simulink model "INTEGRATION_TEST_01"  (Simulink 8.1)
settings: Solver=ode4  StartTime=0.0  StopTime=inf  FixedStep=Ts  MaxStep=1e-3  RelTol=1e-3
model workspace (MAT data in the model file):
  op_snapshot1 : opcond.OperatingPoint (value not decoded)
PostLoadFcn:
  | INTEGRATION_TEST_01_init;
InitFcn:
  | INTEGRATION_TEST_01_init;
values from neighbouring files (symbols this model uses):
  SIM_HIL = 0    [INTEGRATION_TEST_01_init.m]
  Ts = 100E-6    (= 0.0001)    [INTEGRATION_TEST_01_init.m]
undefined symbols (not defined in the file or in its folder): cable_spec, cb_mech_delay, fdesignblkfcn, gcbh, Left, NG_CHP, NG_CHP_lib, ph, relay_par, type, V
libraries: simulink x23, rtio_opalrt_common x21, rtlab x7, simulink_extras x7, cables_lib x6, breaker_lib x4, rteventslib x4, Load_lib x3, rtio_generic_modbus x3, powerlib x2, ssn_lib x2, transformer_lib x2
(part 1 of 2)
settings Model: ARTEMISmethode_block_infos=$$__separator__$$INTEGRATION_TEST_01/ARTEMIS Guide$$__separator__$$  Creator=RE25624  LastModifiedBy=re25624  BufferReuse=off
settings SolverCC: ZeroCrossAlgorithm=Adaptive
settings DataIOCC: ExternalInput=getinputstruct(op_snapshot1)  InitialState=getstatestruct(op_snapshot1)  LimitDataPoints=off  MaxDataPoints=90060  SignalLoggingSaveFormat=Dataset  SaveOutput=off  SignalLogging=off  DSMLogging=off  SaveTime=off  OutputSaveName=result
settings OptimizationCC: BlockReduction=off  OptimizeBlockIOStorage=off  BufferReuse=off  ExpressionFolding=off  LocalBlockOutputs=off
settings DebuggingCC: MaxConsecutiveZCsMsg=warning  IgnoredZcDiagnostic=none  SolverPrmCheckMsg=none  MultiTaskRateTransMsg=warning  FcnCallInpInsideContextMsg=EnableAllAsWarning  FrameProcessingCompatibilityMsg=error  ModelReferenceExtraNoncontSigs=warning  StrictBusMsg=None
settings ModelReferenceCC: UpdateModelReferenceTargets=IfOutOfDate
settings SFSimCC: SFSimEcho=off
settings GRTTargetCC: CodeReplacementLibrary=C89/C90 (ANSI)

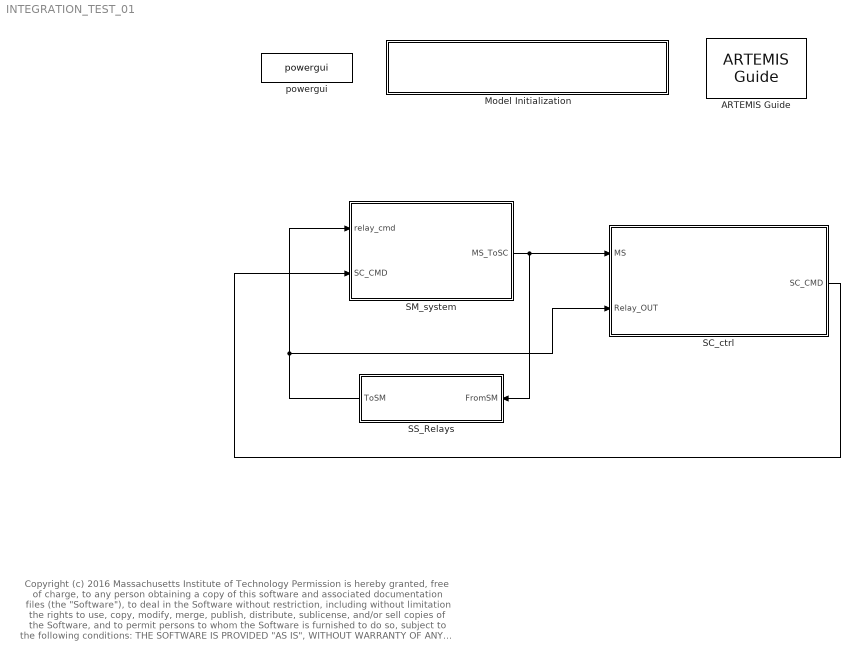
== system INTEGRATION_TEST_01 ==
  note: Copyright (c) 2016 Massachusetts Institute of Technology
      | Permission is hereby granted, free of charge, to any person obtaining a copy of this software and associated documentation files (the "Software"), to deal
      | in the Software without restriction, including without limitation the rights to use, copy, modify, merge, publish, distribute, sublicense, and/or sell copies of the
      | Software, and to permit persons to whom the Software is furnished to do so, subject to the following conditions:
      |
      | THE SOFTWARE IS PROVIDED "AS IS", WITHOUT WARRANTY OF ANY KIND, EXPRESS OR IMPLIED, INCLUDING BUT NOT LIMITED TO THE
      | WARRANTIES OF MERCHANTABILITY, FITNESS FOR A PARTICULAR PURPOSE AND NONINFRINGEMENT. IN NO EVENT SHALL THE AUTHORS
      | OR COPYRIGHT HOLDERS BE LIABLE FOR ANY CLAIM, DAMAGES OR OTHER LIABILITY, WHETHER IN AN ACTION OF CONTRACT, TORT OR
      | OTHERWISE, ARISING FROM, OUT OF OR IN CONNECTION WITH THE SOFTWARE OR THE USE OR OTHER DEALINGS IN THE SOFTWARE.
  ARTEMIS Guide : artemis/ARTEMIS/ARTEMIS Guide  Tag=FTSSmethode_opal_4hx0r99  Description=5.0_z1  lock=on  Ts=Ts  opt=art5  dyna=off  nb_perm=4  RT_fullcomp=off  ssn=on  ssn_itvc=off  ssn_ivic=off  ssn_ext=off  ssn_solver=Art5 with Backward Euler nodal interface  ssn_impulse=off  ssn_quasimpulse=off  ssn_impulse_loop=2  paraExtinctionThy=off  Thy_Impulse=on  dtc=Off  dtc_opt=normal  ao=on  simtype=off  ct_mac=off  lin_mov=off  lsp=[0.001 2]  spike_skip=Disabled  dtc_extra=1  dtc_sws=normal  dtc_pied=0.5  SPSRulesBlock=SPSRules  tre=on  ctmm=off  LF=off  dpl_type=ARTEMiS DPL  rlc_type=off  custom_type=off  para=on  ssn_ImpulseLoopBlockedStateUpdate=2  ssn_mov_iter_number=5  ssn_switch_iter_number=5
  Model Initialization : Subsystem  AncestorBlock=artemis/Tools /Misc/Model Initialization  mask(Model Functions){InitFcnX=INTEGRATION_TEST_01_init;, prel=off, posl=on, inif=on, strf=off}
      mask prompts: InitFcnX "Initialisation"; prel "Preload Function"; posl "PostLoad Function"; inif "InitFcn"; strf "StartFcn"
      mask init:
      | currentBlock = gcb;
      | root = bdroot(currentBlock);
      | 
      | 
      | if ~strcmp(get_param(root,'BlockDiagramType'),'library')
      |     if prel==1
      |         set_param(root, 'PreLoadFcn', InitFcnX);
      |     else
      |         set_param(root, 'PreLoadFcn', '');
      |     end
      |     if inif==1
      |         set_param(root, 'InitFcn', InitFcnX);
      |     else
      |         set_param(root, 'InitFcn', '');
      |     end
      |     if strf==1
      |         set_param(root, 'StartFcn', InitFcnX);
      |     else
      |         set_param(root, 'StartFcn', '');
      |     end
      |     if posl==1
      |         set_param(root, 'PostLoadFcn', InitFcnX);
      |     else
      |         set_param(root, 'PostLoadFcn', '');
      |     end
      | end
      | 
      | pos = get_param(currentBlock, 'Position');
      | width = pos(3) - pos(1); height = pos(4) - pos(2);
      | txt = [ upper(root) '\n' '- InitFcn. . . . . '  get_param(root, 'InitFcn') ];
      settings: CopyFcn=set_param(gcb,'LinkStatus','inactive')
      mask Display: text(5, height*0.5, txt, 'horizontalAlignment', 'left', 'verticalAlignment', 'middle') ;
  SC_ctrl : Subsystem
  SM_system : Subsystem
  SS_Relays : Subsystem
  powergui : powerlib/powergui  Priority=2  SimulationMode=Discrete  SolverType=Tustin  SampleTime=Ts  frequency=60  SPID=off  DisableSnubberDevices=off  DisableRonSwitches=off  DisableVfSwitches=off  SwTol=0  Interpol=off  DisplayEquations=off  frequencyindice=0  Pbase=100e6  ErrMax=1e-4  Iterations=50  UnitsV=kV  UnitsW=MW  FunctionMessages=off  echomessages=off  HookPort=off  EnableUseOfTLC=off  x0status=blocks  RestoreLinks=warning  ResistiveCurrentMeasurement=off  Frange=logspace(0,3,50)  Ylog=off  Xlog=off  ShowGrid=off  save=off  variable=ZData  structure=0  ZoomFFT=on  StartTime=0.0  cycles=2  DisplayStyle=off  fundamental=60  FreqAxis=off  MaxFrequency=1000  frequencyindicesteady=1  RmsSteady=1  display=off  Ts=0  methode=off
  wires:
  SM_system/1(MS_ToSC) -> SC_ctrl/1(MS), SS_Relays/1(FromSM)
  SS_Relays/1(ToSM) -> SM_system/1(relay_cmd), SC_ctrl/2(Relay_OUT)
  SC_ctrl/1(SC_CMD) -> SM_system/2(SC_CMD)

== system INTEGRATION_TEST_01/Model Initialization ==

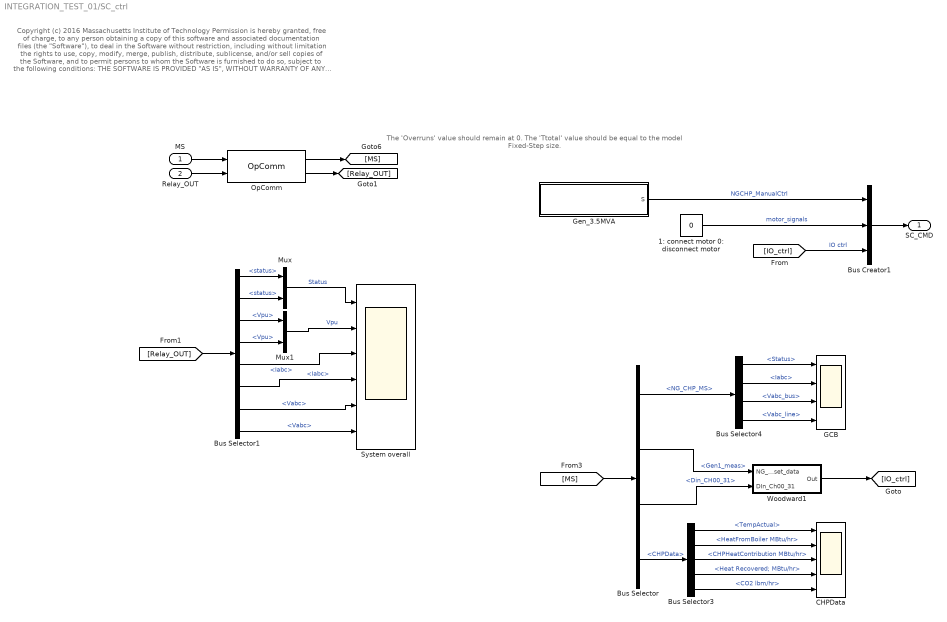
== system INTEGRATION_TEST_01/SC_ctrl ==
  note: The 'Overruns' value should remain at 0.
      | The 'Ttotal' value should be equal to the
      | model Fixed-Step size.
  note: Copyright (c) 2016 Massachusetts Institute of Technology
      | Permission is hereby granted, free of charge, to any person obtaining a copy of this software and associated documentation files (the "Software"), to deal
      | in the Software without restriction, including without limitation the rights to use, copy, modify, merge, publish, distribute, sublicense, and/or sell copies of the
      | Software, and to permit persons to whom the Software is furnished to do so, subject to the following conditions:
      |
      | THE SOFTWARE IS PROVIDED "AS IS", WITHOUT WARRANTY OF ANY KIND, EXPRESS OR IMPLIED, INCLUDING BUT NOT LIMITED TO THE
      | WARRANTIES OF MERCHANTABILITY, FITNESS FOR A PARTICULAR PURPOSE AND NONINFRINGEMENT. IN NO EVENT SHALL THE AUTHORS
      | OR COPYRIGHT HOLDERS BE LIABLE FOR ANY CLAIM, DAMAGES OR OTHER LIABILITY, WHETHER IN AN ACTION OF CONTRACT, TORT OR
      | OTHERWISE, ARISING FROM, OUT OF OR IN CONNECTION WITH THE SOFTWARE OR THE USE OR OTHER DEALINGS IN THE SOFTWARE
  MS : Inport
  Relay_OUT : Inport  Port=2
  1: connect motor 0: disconnect motor : Constant  Value=0
  Bus Creator1 : BusCreator  Inputs=3
  Bus Selector : BusSelector  OutputSignals=NG_CHP_MS,NG_CHP_MS.Gen1_meas,NG_CHP_MS.Din_CH00_31,NG_CHP_MS.CHPData
  Bus Selector1 : BusSelector  OutputSignals=CB2.m.status,CB3.m.status,CB2.m.Vpu,CB3.m.Vpu,CB2.m.Iabc,CB3.m.Iabc,CB2.m.Vabc,CB3.m.Vabc
  Bus Selector3 : BusSelector  OutputSignals=TempActual,HeatFromBoiler MBtu/hr,CHPHeatContribution MBtu/hr,Thermal data.Heat Recovered; MBtu/hr,Thermal data.CO2 lbm/hr
  Bus Selector4 : BusSelector  OutputSignals=NG_CHP_MS.Status,NG_CHP_MS.Iabc,NG_CHP_MS.Vabc_bus,NG_CHP_MS.Vabc_line
  CHPData : Scope  NumInputPorts=5
      settings: ShowLegends=on  TimeRange=10  YMin=20~0~-1~1.37518~932.98  YMax=20.05~5.5~1~1.37533~933.08  SaveName=ScopeData5
  GCB : Scope  NumInputPorts=4
      settings: ShowLegends=on  TimeRange=0.02  YMin=0.95~-800~-100000~-100000  YMax=1.05~800~130000~130000
  Gen_3.5MVA : Subsystem
  Mux : Mux  Inputs=2
  Mux1 : Mux  Inputs=2
  OpComm : rtlab/OpComm  nbport=2  groupe_acq=1  subsys_rate=0  st=0  Synchronization=on  Interpolation=on  Threshold=1.0  Missed_Data=off  Sim_Time=off  Samples=off  dynSigOut=off  from_console=0  warning_done=off  writeOpCommFile=off  Offset=off
  System overall : Scope  NumInputPorts=6
      settings: ShowLegends=on  TimeRange=1  YMin=0~0~-100~-200~-20000~-20000  YMax=5~1.5~100~200~20000~20000
  Woodward1 : Subsystem
  SC_CMD : Outport
  wires:
  OpComm/1 -> [MS]
  MS/1 -> OpComm/1
  OpComm/2 -> [Relay_OUT]
  Relay_OUT/1 -> OpComm/2
  Woodward1/1(Out) -> [IO_ctrl]
  Bus Selector4/1 -> GCB/1  "<Status>"
  Bus Selector4/2 -> GCB/2  "<Iabc>"
  Bus Selector4/3 -> GCB/3  "<Vabc_bus>"
  Bus Selector4/4 -> GCB/4  "<Vabc_line>"
  Bus Selector/1 -> Bus Selector4/1  "<NG_CHP_MS>"
  Bus Selector/2 -> Woodward1/1(NG_genset_data)  "<Gen1_meas>"
  Bus Selector/3 -> Woodward1/2(DIn_Ch00_31)  "<Din_CH00_31>"
  [MS] -> Bus Selector/1
  Bus Selector/4 -> Bus Selector3/1  "<CHPData>"
  Bus Selector3/1 -> CHPData/1  "<TempActual>"
  Bus Selector3/5 -> CHPData/5  "<CO2 lbm/hr>"
  Bus Selector3/2 -> CHPData/2  "<HeatFromBoiler MBtu/hr>"
  Bus Selector3/3 -> CHPData/3  "<CHPHeatContribution MBtu/hr>"
  Bus Selector3/4 -> CHPData/4  "<Heat Recovered; MBtu/hr>"
  [Relay_OUT] -> Bus Selector1/1
  Mux/1 -> System overall/1  "Status"
  Bus Selector1/1 -> Mux/1  "<status>"
  Bus Selector1/2 -> Mux/2  "<status>"
  Bus Selector1/3 -> Mux1/1  "<Vpu>"
  Bus Selector1/4 -> Mux1/2  "<Vpu>"
  Bus Selector1/5 -> System overall/3  "<Iabc>"
  Bus Selector1/6 -> System overall/4  "<Iabc>"
  Bus Selector1/7 -> System overall/5  "<Vabc>"
  Bus Selector1/8 -> System overall/6  "<Vabc>"
  Mux1/1 -> System overall/2  "Vpu"
  Bus Creator1/1 -> SC_CMD/1
  1: connect motor 0: disconnect motor/1 -> Bus Creator1/2  "motor_signals"
  [IO_ctrl] -> Bus Creator1/3  "IO ctrl"
  Gen_3.5MVA/1(S) -> Bus Creator1/1  "NGCHP_ManualCtrl"

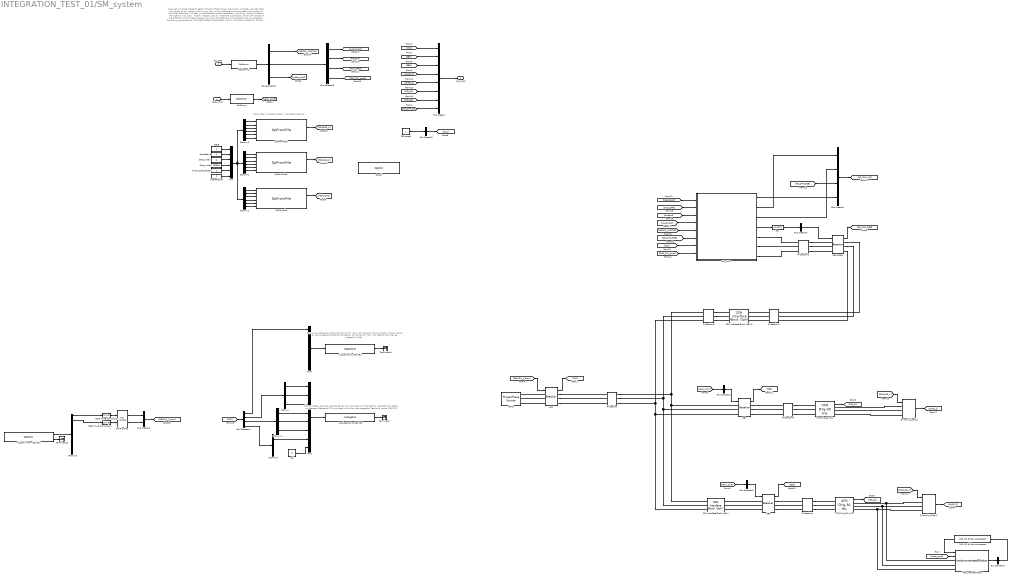
== system INTEGRATION_TEST_01/SM_system ==
  note: Copyright (c) 2016 Massachusetts Institute of Technology
      | Permission is hereby granted, free of charge, to any person obtaining a copy of this software and associated documentation files (the "Software"), to deal
      | in the Software without restriction, including without limitation the rights to use, copy, modify, merge, publish, distribute, sublicense, and/or sell copies of the
      | Software, and to permit persons to whom the Software is furnished to do so, subject to the following conditions:
      |
      | THE SOFTWARE IS PROVIDED "AS IS", WITHOUT WARRANTY OF ANY KIND, EXPRESS OR IMPLIED, INCLUDING BUT NOT LIMITED TO THE
      | WARRANTIES OF MERCHANTABILITY, FITNESS FOR A PARTICULAR PURPOSE AND NONINFRINGEMENT. IN NO EVENT SHALL THE AUTHORS
      | OR COPYRIGHT HOLDERS BE LIABLE FOR ANY CLAIM, DAMAGES OR OTHER LIABILITY, WHETHER IN AN ACTION OF CONTRACT, TORT OR
      | OTHERWISE, ARISING FROM, OUT OF OR IN CONNECTION WITH THE SOFTWARE OR THE USE OR OTHER DEALINGS IN THE SOFTWARE
  note: Stop_index = length of data - 1 to data chopping
  note: This connector also services Genset #2 and  is
      | shared with Genset #1.  Use RJ45 connectors to
      |  intercept Genset #2 I/O (not used in this Device
      | Integration Test) and use for SEL-751
  note: Remove existing connections to Slot 3 I/O, if any
      | ans replace with connections shown below, or use
      | corresponding RJ45 connectors.  (Existing I/O, if any not
      |  used for this Device Integration Test)
  relay_cmd : Inport
  SC_CMD : Inport  Port=2
  200 HP chiller compressor : Load_lib/200 HP chiller compressor
  AnalogOut2 to SEL-751 : rtio_opalrt_common/AnalogOut  CtrlName='OpCtrl'  portNb=4  FcnNos=Slot 2 Module A Subsection 2  size=16  maxcount=8  count=8  numchan=8  israngeinput=off  voltagerange=[ -5 ... 5 ]  slot=1  side=0  mismatch=0  slotside=Slot_2_Module_A
      settings: AttributesFormatString=%<CtrlName>
  Bus Creator : BusCreator  Inputs=8
  Bus Creator1 : BusCreator
  Bus Creator2 : BusCreator  Inputs=1
  Bus Creator3 : BusCreator  Inputs=1
  Bus Creator4 : BusCreator  Inputs=2
  Bus Selector1 : BusSelector  OutputSignals=CB2
  Bus Selector2 : BusSelector  OutputSignals=CB3
  Bus Selector3 : BusSelector  OutputSignals=NGCHP_ManualCtrl,IO ctrl,motor_signals
  Bus Selector4 : BusSelector  OutputSignals=Status,Iabc,Vabc_line,Vabc_bus
  Bus Selector5 : BusSelector  OutputSignals=Woodward,manual_controls,DOUT GR3,DOUT GR3.16 DOUT GR3.CHP_SIM_Cmds
  Bus Selector6 : BusSelector  OutputSignals=RPM
  CB closed : Constant
  CB1-GCB1 : breaker_lib/Breaker  Ts=Ts  mech_delays=[cb_mech_delay(1,:)]
  CB2 : breaker_lib/Breaker  Ts=Ts  mech_delays=[cb_mech_delay(1,:)]
  CB3 : breaker_lib/Breaker  Ts=Ts  mech_delays=[cb_mech_delay(1,:)]
  Cal : Constant  Value=0
  Data Type Conversion : DataTypeConversion
  Data Type Conversion1 : DataTypeConversion
  Demux : Demux  Outputs=3
  Demux1 : Demux  Outputs=6
  Demux2 : Demux  Outputs=6
  Demux3 : Demux  Outputs=6
  Demux4 : Demux  Outputs=3
  Demux5 : Demux  Outputs=3
  Demux6 : Demux  Outputs=8
  DigitalIn from SEL-751 : rtio_opalrt_common/DigitalIn  CtrlName='OpCtrl'  portNb=6  FcnNos=Slot 3 Module A Subsection 2  size=1  maxcount=8  count=8  sampleTime=Ts  numchan=8
      settings: AttributesFormatString=%<CtrlName>
  DigitalOut to SEL-751 : rtio_opalrt_common/DigitalOut  CtrlName='OpCtrl'  portNb=6  FcnNos=Slot 3 Module B Subsection 2  size=1  maxcount=8  count=8  numchan=8
      settings: AttributesFormatString=%<CtrlName>
  Dynamic_Load_1 : Load_lib/Dynamic_Load  V=4160  Ts=Ts
  Dynamic_Load_2 : Load_lib/Dynamic_Load  V=480  Ts=Ts
  Fcn : Fcn  Expr=u(1)==1
  GRID : powerlib/Electrical Sources/Three-Phase Source  Voltage=13800  PhaseAngle=0  Frequency=60  InternalConnection=Yg  SpecifyImpedance=on  Resistance=0.8929  Inductance=16.58e-3  ShortCircuitLevel=375e6  BaseVoltage=13800  XRratio=4.6  BusType=swing  Pref=0  Qref=0  Qmin=-inf  Qmax=inf
  InstrumentedMotor : Motor_InductionMachine_lib/InstrumentedMotor
  "Interpolation " : Constant
  MID : breaker_lib/Breaker  Ts=Ts  mech_delays=[cb_mech_delay(1,:)]
  Mux : Mux  Inputs=6
  Mux1 : Mux  Inputs=8
  Mux4 : Mux  Inputs=8
  NG_CHP1 : Subsystem  AncestorBlock=NG_CHP_lib/NG_CHP
  OpComm : rtlab/OpComm  nbport=1  groupe_acq=1  subsys_rate=0  st=0  Synchronization=on  Interpolation=on  Threshold=1.0  Missed_Data=off  Sim_Time=off  Samples=off  dynSigOut=off  from_console=0  warning_done=off  writeOpCommFile=off  Offset=off
  OpComm2 : rtlab/OpComm  nbport=1  groupe_acq=1  subsys_rate=0  st=0  Synchronization=on  Interpolation=on  Threshold=1.0  Missed_Data=off  Sim_Time=off  Samples=off  dynSigOut=off  from_console=1  warning_done=off  writeOpCommFile=off  Offset=off
  OpCtrl : rtio_opalrt_common/OpCtrl  CtrlName='OpCtrl'  boardid=0  BitstreamFilename=VC707_2-EX-0001-2_2_6_61-32AIO16DIO16DIOSel-01-01.bin  numconfig=-1  mode=Master  externalClock=off  decimRtsi=0  calibIO=off  SampleTime=0  loadinport=-1  BoardType=VC707  SecondaryPresent=off  sync_type=Audio
  OpFromFile : rtlab/DataLogging/OpFromFile  filename_mode=Static (same filename all the time)  reload_mode=Next time model is paused (Real-Time)  init_file_id=0  filename=HeatLoad.mat  rtpath='./'  nrtpath='.\'  sample_time=Ts
  OpFromFile1 : rtlab/DataLogging/OpFromFile  filename_mode=Static (same filename all the time)  reload_mode=Next time model is paused (Real-Time)  init_file_id=0  filename=one_min_data.mat  rtpath='./'  nrtpath='.\'  sample_time=0
  OpFromFile2 : rtlab/DataLogging/OpFromFile  filename_mode=Static (same filename all the time)  reload_mode=Next time model is paused (Real-Time)  init_file_id=0  filename=one_min_data.mat  rtpath='./'  nrtpath='.\'  sample_time=0
  PI-Section : cables_lib/PI-Section  cable_spec=[cable_spec(13, :)]  line_length=5500  parallel_sets=1
  PI-Section1 : cables_lib/PI-Section  cable_spec=[cable_spec(11, :)]  line_length=10  parallel_sets=1
  PI-Section2 : cables_lib/PI-Section  cable_spec=[cable_spec(11, :)]  line_length=2000  parallel_sets=1
  PI-Section3 : cables_lib/PI-Section  cable_spec=[cable_spec(13, :)]  line_length=1500  parallel_sets=1
  PI-Section4 : cables_lib/PI-Section  cable_spec=[cable_spec(13, :)]  line_length=7000  parallel_sets=1
  PI-Section5 : cables_lib/PI-Section  cable_spec=[cable_spec(11, :)]  line_length=10  parallel_sets=1
  "Repetative " : Constant
  S-R Flip-Flop : simulink_extras/Flip Flops/S-R Flip-Flop  initial_condition=1
  SSN Interface Block (3ph) : ssn_lib/SSN Interface Block (3ph)  nb_phase=3  nb_port=2  p1_type=V-type(Left)  p2_type=V-type (Right)  p3_type=V-type(Left)  p4_type=V-type(Left)  p5_type=V-type(Left)  p6_type=V-type(Left)  p7_type=V-type(Left)  p8_type=V-type(Left)  p9_type=V-type(Left)  p10_type=V-type(Left)  p11_type=V-type(Left)  p12_type=V-type(Left)  p13_type=V-type(Left)  p14_type=V-type(Left)  p15_type=V-type(Left)  p16_type=V-type(Left)  I_port_shunt_resistance=1e9
  SSN Interface Block (3ph)1 : ssn_lib/SSN Interface Block (3ph)  nb_phase=3  nb_port=2  p1_type=V-type(Left)  p2_type=V-type (Right)  p3_type=V-type(Left)  p4_type=V-type(Left)  p5_type=V-type(Left)  p6_type=V-type(Left)  p7_type=V-type(Left)  p8_type=V-type(Left)  p9_type=V-type(Left)  p10_type=V-type(Left)  p11_type=V-type(Left)  p12_type=V-type(Left)  p13_type=V-type(Left)  p14_type=V-type(Left)  p15_type=V-type(Left)  p16_type=V-type(Left)  I_port_shunt_resistance=1e9
  "Start_Index " : Constant
  "State " : Constant
  "Stop_Index " : Constant  Value=1800-1
  Terminator : Terminator
  Terminator1 : Terminator
  Terminator2 : Terminator
  "Time_Scale_Factor " : Constant
  XFR DYg-30 HIL1 : transformer_lib/XFR DYg-30 HIL  Rating=3750  Vp=13800  Vs=4160  Z=4.75  XR=11.4
  XFR DYg-30 HIL2 : transformer_lib/XFR DYg-30 HIL  Rating=2500  Vp=13800  Vs=480  Z=5.75  XR=6.6
  MS_ToSC : Outport
  wires:
  MID/1 -> [MID]
  Bus Creator/1 -> MS_ToSC/1
  OpComm/1 -> [relay_cmd]
  relay_cmd/1 -> OpComm/1
  CB1-GCB1/1 -> [NG_CHP_GCB]
  SC_CMD/1 -> OpComm2/1
  Bus Selector5/1 -> [woodward]  "<Woodward>"
  Bus Selector5/3 -> [Dout_GR3]  "<DOUT GR3>"
  Bus Selector5/2 -> [brkcont]  "<manual_controls>"
  [NG_CHP_GCB] -> Bus Creator1/3  "NG_CHP_MS"
  NG_CHP1/3(Generator Data) -> Bus Creator1/2  "Gen1_meas"
  NG_CHP1/2(Out2) -> Bus Creator1/1  "Din_CH00_31"
  XFR DYg-30 HIL1/1 -> [XFR_01]
  "Stop_Index "/1 -> Mux/4
  Demux1/2 -> OpFromFile1/2
  Demux1/5 -> OpFromFile1/5
  OpFromFile1/2 -> [PQLOAD_2]
  "Interpolation "/1 -> Mux/6
  Demux1/4 -> OpFromFile1/4
  Demux1/1 -> OpFromFile1/1
  Demux1/6 -> OpFromFile1/6
  Demux1/3 -> OpFromFile1/3
  "Start_Index "/1 -> Mux/3
  "Time_Scale_Factor "/1 -> Mux/5
  "Repetative "/1 -> Mux/2
  "State "/1 -> Mux/1
  [Dout_GR3] -> NG_CHP1/2(Digital Outputs)
  [brkcont] -> NG_CHP1/3(Console Breakers)
  [woodward] -> NG_CHP1/4(Woodward Enable)
  [NGCHP_MNCTLR] -> NG_CHP1/5(Manual Control (opt))
  [NG_CHP_GCB] -> NG_CHP1/6(GCB)
  [MID] -> NG_CHP1/7(MCB)
  NG_CHP1/1(Out1) -> Bus Creator1/4  "CHPData"
  NG_CHP1/4(GCB Control) -> Fcn/1
  Bus Selector5/4 -> [CHP_SIM_cmds]  "<CHP_SIM_Cmds>"
  OpFromFile/2 -> [heat_load]  "Heat Load MBtu/hr"
  [heat_load] -> NG_CHP1/1(In1)
  [CHP_SIM_cmds] -> NG_CHP1/8(In2)
  Demux2/2 -> OpFromFile/2
  Demux2/5 -> OpFromFile/5
  Demux2/4 -> OpFromFile/4
  Demux2/1 -> OpFromFile/1
  Demux2/6 -> OpFromFile/6
  Demux2/3 -> OpFromFile/3
  Dynamic_Load_1/1 -> [LOAD_1]
  XFR DYg-30 HIL2/1 -> [XFR_02]
  Dynamic_Load_2/1 -> [LOAD_2]
  Bus Creator2/1 -> [cb_c]
  CB closed/1 -> Bus Creator2/1  "Logic_trip"
  CB2/1 -> [CB2]
  CB3/1 -> [CB3]
  [XFR_02] -> Bus Creator/7  "XFR_02"
  [LOAD_2] -> Bus Creator/5  "LOAD_2"
  [XFR_01] -> Bus Creator/6  "XFR_01"
  [MID] -> Bus Creator/1  "MID"
  [CB3] -> Bus Creator/3  "CB3"
  [CB2] -> Bus Creator/2  "CB2"
  [LOAD_1] -> Bus Creator/4  "LOAD_1"
  Bus Creator1/1 -> [NG_CHP_MS]
  [NG_CHP_MS] -> Bus Creator/8  "NG_CHP_MS"
  Demux3/2 -> OpFromFile2/2
  Demux3/5 -> OpFromFile2/5
  OpFromFile2/2 -> [PQLOAD_1]
  Demux3/4 -> OpFromFile2/4
  Demux3/1 -> OpFromFile2/1
  Demux3/6 -> OpFromFile2/6
  Demux3/3 -> OpFromFile2/3
  Mux/1 -> Demux3/1, Demux2/1, Demux1/1
  [PQLOAD_1] -> Dynamic_Load_1/1
  [PQLOAD_2] -> Dynamic_Load_2/1
  [relay_cmd] -> Bus Selector1/1
  Bus Selector1/1 -> CB2/1  "<CB2>"
  [relay_cmd] -> Bus Selector2/1
  Bus Selector2/1 -> CB3/1  "<CB3>"
  Fcn/1 -> Bus Creator3/1  "Logic_trip"
  Bus Creator3/1 -> CB1-GCB1/1  "Logic_trip"
  [SEL751_1_from] -> MID/1
  [motor_cmd] -> InstrumentedMotor/2
  InstrumentedMotor/1 -> Bus Selector6/1
  Bus Selector6/1 -> 200 HP chiller compressor/1  "<RPM>"
  200 HP chiller compressor/1 -> InstrumentedMotor/1
  OpComm2/1 -> Bus Selector3/1
  Bus Selector3/1 -> [NGCHP_MNCTLR]  "<NGCHP_ManualCtrl>"
  Bus Selector3/2 -> Bus Selector5/1  "<IO ctrl>"
  Bus Selector3/3 -> [motor_cmd]  "<motor_signals>"
  Bus Selector4/2 -> Demux/1  "<Iabc>"
  Demux4/1 -> Mux1/4  "Va"
  Demux4/2 -> Mux1/5  "Vb"
  Demux4/3 -> Mux1/6  "Vc"
  Bus Selector4/4 -> Demux5/1  "<Vabc_bus>"
  Demux5/1 -> Mux1/7  "Vs"
  Bus Selector4/3 -> Demux4/1  "<Vabc_line>"
  Cal/1 -> Mux1/8
  AnalogOut2 to SEL-751/1 -> Terminator/1
  DigitalIn from SEL-751/1 -> Demux6/1
  Demux6/1 -> Data Type Conversion/1  "OUT103 Brkr trip"
  Demux6/2 -> Data Type Conversion1/1  "OUT102 Brkr reset"
  Data Type Conversion/1 -> S-R Flip-Flop/1
  Data Type Conversion1/1 -> S-R Flip-Flop/2
  S-R Flip-Flop/1 -> Bus Creator4/1  "Logic_trip"
  S-R Flip-Flop/2 -> Bus Creator4/2  "Logic_reset"
  Bus Selector4/1 -> Mux4/1  "<Status>"
  Mux4/1 -> DigitalOut to SEL-751/1
  DigitalOut to SEL-751/1 -> Terminator1/1
  DigitalIn from SEL-751/2 -> Terminator2/1
  Mux1/1 -> AnalogOut2 to SEL-751/1
  Demux/1 -> Mux1/1  "Ia"
  Demux/3 -> Mux1/3  "Ic"
  Demux/2 -> Mux1/2  "Ib"
  Bus Creator4/1 -> [SEL751_1_from]
  [MID] -> Bus Selector4/1
  connections:
  Dynamic_Load_1/LConn1 -- XFR DYg-30 HIL1/RConn1
  Dynamic_Load_1/LConn2 -- XFR DYg-30 HIL1/RConn2
  Dynamic_Load_1/LConn3 -- XFR DYg-30 HIL1/RConn3
  CB2/RConn2 -- PI-Section3/LConn2
  CB2/RConn1 -- PI-Section3/LConn1
  CB2/RConn3 -- PI-Section3/LConn3
  CB3/RConn2 -- PI-Section4/LConn2
  CB3/RConn1 -- PI-Section4/LConn1
  CB3/RConn3 -- PI-Section4/LConn3
  CB3/LConn2 -- SSN Interface Block (3ph)/RConn2
  CB3/LConn1 -- SSN Interface Block (3ph)/RConn1
  CB3/LConn3 -- SSN Interface Block (3ph)/RConn3
  PI-Section5/LConn3 -- PI-Section/RConn3 -- SSN Interface Block (3ph)/LConn3 -- CB2/LConn3
  PI-Section5/LConn2 -- PI-Section/RConn2 -- SSN Interface Block (3ph)/LConn2 -- CB2/LConn2
  PI-Section5/LConn1 -- PI-Section/RConn1 -- SSN Interface Block (3ph)/LConn1 -- CB2/LConn1
  Dynamic_Load_2/LConn1 -- InstrumentedMotor/LConn1 -- XFR DYg-30 HIL2/RConn1
  Dynamic_Load_2/LConn3 -- InstrumentedMotor/LConn3 -- XFR DYg-30 HIL2/RConn3
  Dynamic_Load_2/LConn2 -- InstrumentedMotor/LConn2 -- XFR DYg-30 HIL2/RConn2
  PI-Section4/RConn1 -- XFR DYg-30 HIL2/LConn1
  PI-Section4/RConn2 -- XFR DYg-30 HIL2/LConn2
  PI-Section4/RConn3 -- XFR DYg-30 HIL2/LConn3
  PI-Section3/RConn2 -- XFR DYg-30 HIL1/LConn2
  PI-Section3/RConn3 -- XFR DYg-30 HIL1/LConn3
  PI-Section3/RConn1 -- XFR DYg-30 HIL1/LConn1
  PI-Section2/RConn3 -- CB1-GCB1/LConn3
  PI-Section2/RConn2 -- CB1-GCB1/LConn2
  PI-Section2/RConn1 -- CB1-GCB1/LConn1
  NG_CHP1/RConn2 -- PI-Section2/LConn2
  NG_CHP1/RConn3 -- PI-Section2/LConn3
  NG_CHP1/RConn1 -- PI-Section2/LConn1
  PI-Section1/LConn1 -- SSN Interface Block (3ph)1/RConn1
  PI-Section1/LConn2 -- SSN Interface Block (3ph)1/RConn2
  PI-Section1/LConn3 -- SSN Interface Block (3ph)1/RConn3
  PI-Section5/RConn2 -- SSN Interface Block (3ph)1/LConn2
  PI-Section5/RConn1 -- SSN Interface Block (3ph)1/LConn1
  PI-Section5/RConn3 -- SSN Interface Block (3ph)1/LConn3
  CB1-GCB1/RConn3 -- PI-Section1/RConn3
  CB1-GCB1/RConn1 -- PI-Section1/RConn1
  CB1-GCB1/RConn2 -- PI-Section1/RConn2
  MID/RConn3 -- PI-Section/LConn3
  MID/RConn2 -- PI-Section/LConn2
  MID/RConn1 -- PI-Section/LConn1
  MID/LConn3 -- GRID/RConn3
  MID/LConn1 -- GRID/RConn1
  MID/LConn2 -- GRID/RConn2

== system INTEGRATION_TEST_01/SS_Relays ==
  note: Copyright (c) 2016 Massachusetts Institute of Technology
      | Permission is hereby granted, free of charge, to any person obtaining a copy of this software and associated documentation files (the "Software"), to deal
      | in the Software without restriction, including without limitation the rights to use, copy, modify, merge, publish, distribute, sublicense, and/or sell copies of the
      | Software, and to permit persons to whom the Software is furnished to do so, subject to the following conditions:
      |
      | THE SOFTWARE IS PROVIDED "AS IS", WITHOUT WARRANTY OF ANY KIND, EXPRESS OR IMPLIED, INCLUDING BUT NOT LIMITED TO THE
      | WARRANTIES OF MERCHANTABILITY, FITNESS FOR A PARTICULAR PURPOSE AND NONINFRINGEMENT. IN NO EVENT SHALL THE AUTHORS
      | OR COPYRIGHT HOLDERS BE LIABLE FOR ANY CLAIM, DAMAGES OR OTHER LIABILITY, WHETHER IN AN ACTION OF CONTRACT, TORT OR
      | OTHERWISE, ARISING FROM, OUT OF OR IN CONNECTION WITH THE SOFTWARE OR THE USE OR OTHER DEALINGS IN THE SOFTWARE
  FromSM : Inport
  Bus Creator : BusCreator  Inputs=2
  Bus Selector : BusSelector  OutputSignals=CB2,CB3
  Generic_Relay_v2_1 : relay_modbus_lib/Generic_Relay_v2_1  Ts=Ts  relay_settings=[relay_par(1,:)]
  Generic_Relay_v2_2 : relay_modbus_lib/Generic_Relay_v2_1  Ts=Ts  relay_settings=[relay_par(2,:)]
  Modbus device : rtio_generic_modbus/Modbus device  conf_name=F1_relay_cfg1.opal  conf_name_mask=F1_relay_cfg1.xls  sample_time=Ts
  Modbus device1 : rtio_generic_modbus/Modbus device  conf_name=F1_relay_cfg2.opal  conf_name_mask=F1_relay_cfg2.xls  sample_time=Ts
  OpComm : rtlab/OpComm  nbport=1  groupe_acq=1  subsys_rate=0  st=0  Synchronization=on  Interpolation=on  Threshold=1.0  Missed_Data=off  Sim_Time=off  Samples=off  dynSigOut=off  from_console=0  warning_done=off  writeOpCommFile=off  Offset=off
  ToSM : Outport
  wires:
  OpComm/1 -> Bus Selector/1
  FromSM/1 -> OpComm/1
  Generic_Relay_v2_1/1 -> Bus Creator/1  "CB2"
  Generic_Relay_v2_2/1 -> Bus Creator/2  "CB3"
  Bus Creator/1 -> ToSM/1
  Modbus device/1 -> Generic_Relay_v2_1/2
  Generic_Relay_v2_1/2 -> Modbus device/1
  Modbus device1/1 -> Generic_Relay_v2_2/2
  Generic_Relay_v2_2/2 -> Modbus device1/1
  Bus Selector/2 -> Generic_Relay_v2_2/1  "<CB3>"
  Bus Selector/1 -> Generic_Relay_v2_1/1  "<CB2>"

== system INTEGRATION_TEST_01/SC_ctrl/Gen_3.5MVA ==
  1 - PQ 2 - PV 3 - VF : Constant  Value=3
  2.5 - 130 s : DiscretePulseGenerator  Period=150/Ts  PulseWidth=127.5/Ts  PhaseDelay=2.5/Ts  SampleTime=Ts
  Bus Creator : BusCreator  Inputs=6
  DONOTCHANGE : Constant
  Enable = 1 Disable = 0 : Constant  Value=0
  F : simulink/Math Operations/Slider Gain  low=0.97  gain=1  high=1.03
  Fcmd pu : Constant  Value=1.0
  P : simulink/Math Operations/Slider Gain  low=0  gain=0.8  high=1.1
  Pfactor : Gain  Gain=.9
  Q : simulink/Math Operations/Slider Gain  low=0.01  gain=0.2  high=0.4
  Qfactor : Gain  Gain=.43
  S Profile : simulink/Sources/Repeating Sequence Stair  OutValues=[.1 .1 .1 .1 .1 .1 .5 .5 .5 .5 .5 .5 .5 .5 .5 .5 .5 .5 1 1 1 1 1 ]  tsamp=[5 Ts]  OutMin=[]  OutMax=[]  OutDataTypeStr=Inherit: Inherit via back propagation  OutDataType=fixdt(0,8)  ConRadixGroup=Best Precision: Vector-wise  OutScaling=2^-12
  V : simulink/Math Operations/Slider Gain  low=0.9  gain=1  high=1.1
  VF - to end : simulink/Sources/Repeating Sequence Stair  OutValues=[3 3 3 3 3 3 3 3 3 3 3 3 3 3 3 3 3 3 3 3 3 3 3 3 3 3 3 3 3 3 3 ]  tsamp=[5 Ts]  OutMin=[]  OutMax=[]  OutDataTypeStr=Inherit: Inherit via back propagation  OutDataType=fixdt(0,8)  ConRadixGroup=Best Precision: Vector-wise  OutScaling=2^-12
  Vcmd pu : Constant
  S : Outport
  wires:
  Pfactor/1 -> Bus Creator/1  "P"
  Fcmd pu/1 -> Bus Creator/4  "F"
  2.5 - 130 s/1 -> Bus Creator/6  "Enable"
  VF - to end/1 -> Bus Creator/5  "Mode"
  Vcmd pu/1 -> Bus Creator/3  "V"
  Qfactor/1 -> Bus Creator/2  "Q"
  S Profile/1 -> Pfactor/1, Qfactor/1  "P"
  Bus Creator/1 -> S/1
  DONOTCHANGE/1 -> F/1, V/1, Q/1, P/1

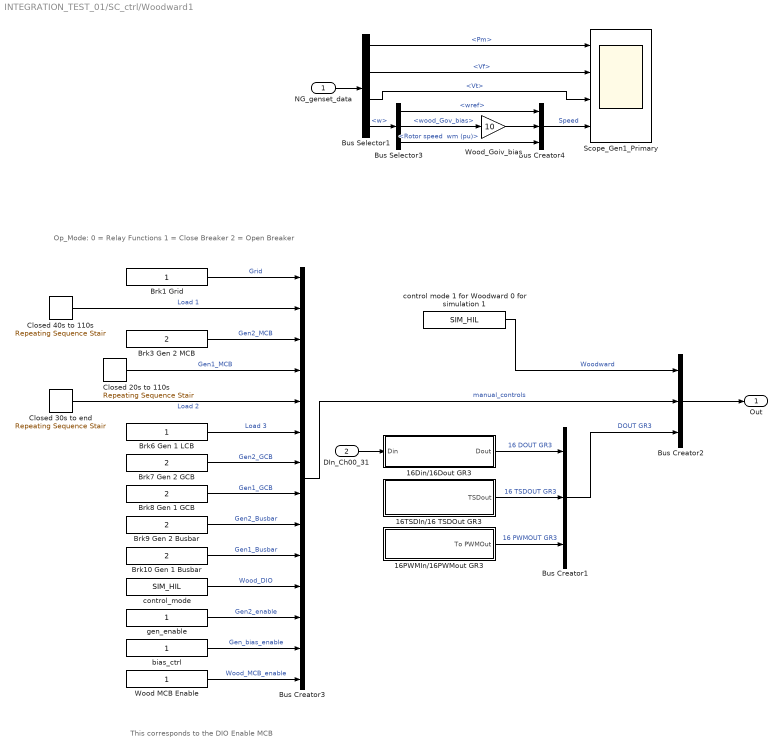
== system INTEGRATION_TEST_01/SC_ctrl/Woodward1 ==
  note: This corresponds to
      | the DIO Enable MCB
  note: Op_Mode:
      | 0 = Relay Functions
      | 1 = Close Breaker
      | 2 = Open Breaker
  NG_genset_data : Inport
  DIn_Ch00_31 : Inport  Port=2
  16Din/16Dout GR3 : Subsystem
  16PWMIn/16PWMout GR3 : Subsystem
  16TSDIn/16 TSDOut GR3 : Subsystem
  Brk1 Grid : Constant
  Brk10 Gen 1 Busbar : Constant  Value=2
  Brk3 Gen 2 MCB : Constant  Value=2
  Brk6 Gen 1 LCB : Constant
  Brk7 Gen 2 GCB : Constant  Value=2
  Brk8 Gen 1 GCB : Constant  Value=2
  Brk9 Gen 2 Busbar : Constant  Value=2
  Bus Creator1 : BusCreator  Inputs=3
  Bus Creator2 : BusCreator  Inputs=3
  Bus Creator3 : BusCreator  Inputs=14
  Bus Creator4 : BusCreator  Inputs=3
  Bus Selector1 : BusSelector  OutputSignals=Pm,Vf,Vt,w
  Bus Selector3 : BusSelector  OutputSignals="wref,w.wood_Gov_bias,w.Rotor speed  wm (pu)"
  Closed 20s to 110s : simulink/Sources/Repeating Sequence Stair  OutValues=[2 2 2 2 1 1 1 1 1 1 1 1 1 1 1 1 1 1 1 1 1 1 2 2 2 2 2]  tsamp=[5 Ts]  OutMin=[]  OutMax=[]  OutDataTypeStr=double  OutputDataTypeScalingMode=double  OutDataType=fixdt(0,8)  ConRadixGroup=Best Precision: Vector-wise  OutScaling=2^-12
  Closed 30s to end : simulink/Sources/Repeating Sequence Stair  OutValues=[2 2 2 2 2 2 1 1 1 1 1 1 1 1 1 1 1 1 1 1 1 1 ]  tsamp=[5 Ts]  OutMin=[]  OutMax=[]  OutDataTypeStr=double  OutputDataTypeScalingMode=double  OutDataType=fixdt(0,8)  ConRadixGroup=Best Precision: Vector-wise  OutScaling=2^-12
  Closed 40s to 110s : simulink/Sources/Repeating Sequence Stair  OutValues=[2 2 2 2 2 2 2 2 1 1 1 1 1 1 1 1 1 1 1 1 1 1 2 2 2]  tsamp=[5 Ts]  OutMin=[]  OutMax=[]  OutDataTypeStr=double  OutputDataTypeScalingMode=double  OutDataType=fixdt(0,8)  ConRadixGroup=Best Precision: Vector-wise  OutScaling=2^-12
  Scope_Gen1_Primary : Scope  NumInputPorts=4
      settings: TimeRange=10  YMin=-0.025~-0.5~0~0  YMax=0.45~5.5~1.1~0.425  SaveName=ScopeData4
  Wood MCB Enable : Constant
  Wood_Goiv_bias : Gain  Gain=10
  bias_ctrl : Constant
  control mode 1 for Woodward 0 for simulation 1 : Constant  Value=SIM_HIL
  control_mode : Constant  Value=SIM_HIL
  gen_enable : Constant
  Out : Outport
  wires:
  Brk1 Grid/1 -> Bus Creator3/1  "Grid"
  Brk10 Gen 1 Busbar/1 -> Bus Creator3/10  "Gen1_Busbar"
  Brk9 Gen 2 Busbar/1 -> Bus Creator3/9  "Gen2_Busbar"
  Wood_Goiv_bias/1 -> Bus Creator4/2
  Brk8 Gen 1 GCB/1 -> Bus Creator3/8  "Gen1_GCB"
  Brk7 Gen 2 GCB/1 -> Bus Creator3/7  "Gen2_GCB"
  Brk6 Gen 1 LCB/1 -> Bus Creator3/6  "Load 3"
  Closed 30s to end/1 -> Bus Creator3/5  "Load 2"
  Bus Creator4/1 -> Scope_Gen1_Primary/4  "Speed"
  Bus Selector3/3 -> Bus Creator4/3  "<Rotor speed  wm (pu)>"
  Bus Selector3/2 -> Wood_Goiv_bias/1  "<wood_Gov_bias>"
  Bus Selector3/1 -> Bus Creator4/1  "<wref>"
  Bus Selector1/4 -> Bus Selector3/1  "<w>"
  Wood MCB Enable/1 -> Bus Creator3/14  "Wood_MCB_enable"
  NG_genset_data/1 -> Bus Selector1/1
  Bus Selector1/3 -> Scope_Gen1_Primary/3  "<Vt>"
  Bus Selector1/2 -> Scope_Gen1_Primary/2  "<Vf>"
  Bus Selector1/1 -> Scope_Gen1_Primary/1  "<Pm>"
  DIn_Ch00_31/1 -> 16Din/16Dout GR3/1(Din)
  Bus Creator2/1 -> Out/1
  bias_ctrl/1 -> Bus Creator3/13  "Gen_bias_enable"
  gen_enable/1 -> Bus Creator3/12  "Gen2_enable"
  control_mode/1 -> Bus Creator3/11  "Wood_DIO"
  Closed 20s to 110s/1 -> Bus Creator3/4  "Gen1_MCB"
  Brk3 Gen 2 MCB/1 -> Bus Creator3/3  "Gen2_MCB"
  Closed 40s to 110s/1 -> Bus Creator3/2  "Load 1"
  Bus Creator3/1 -> Bus Creator2/2  "manual_controls"
  Bus Creator1/1 -> Bus Creator2/3  "DOUT GR3"
  16PWMIn/16PWMout GR3/1(To PWMOut) -> Bus Creator1/3  "16 PWMOUT GR3"
  16TSDIn/16 TSDOut GR3/1(TSDout) -> Bus Creator1/2  "16 TSDOUT GR3"
  16Din/16Dout GR3/1(Dout) -> Bus Creator1/1  "16 DOUT GR3"
  control mode 1 for Woodward 0 for simulation 1/1 -> Bus Creator2/1  "Woodward"

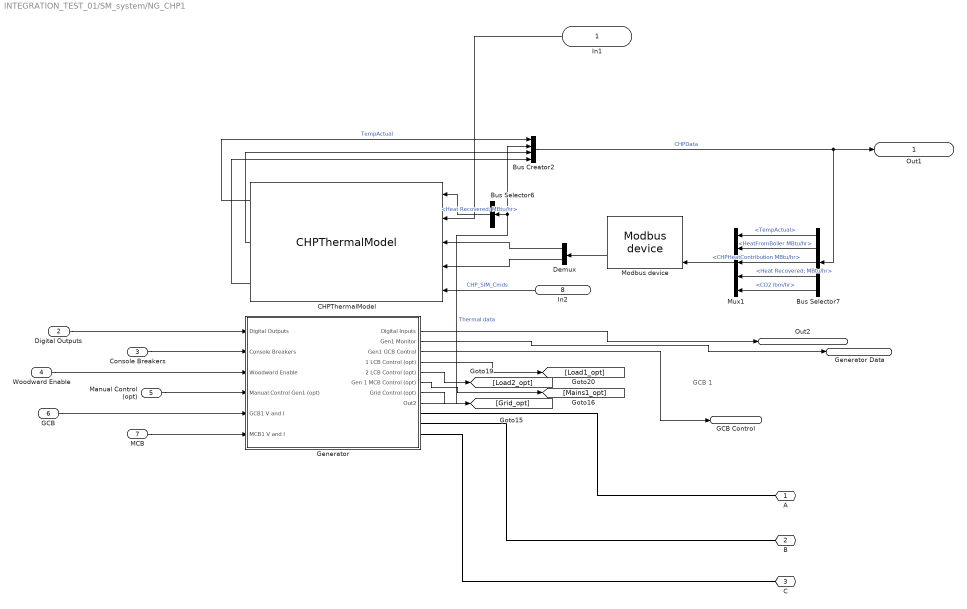
== system INTEGRATION_TEST_01/SM_system/NG_CHP1 ==
  note: GCB 1
  In1 : Inport
  Digital Outputs : Inport  Port=2
  Console Breakers : Inport  Port=3
  Woodward Enable : Inport  Port=4
  Manual Control (opt) : Inport  Port=5
  GCB : Inport  Port=6
  MCB : Inport  Port=7
  In2 : Inport  Port=8
  Bus Creator2 : BusCreator
  Bus Selector6 : BusSelector  OutputSignals=Heat Recovered; MBtu/hr
  Bus Selector7 : BusSelector  OutputSignals=TempActual,HeatFromBoiler MBtu/hr,CHPHeatContribution MBtu/hr,Thermal data.Heat Recovered; MBtu/hr,Thermal data.CO2 lbm/hr
  CHPThermalModel : CHP_Model_lib/CHPThermalModel  SIM_HIL=SIM_HIL
  Demux : Demux  Outputs=2
  Generator : Subsystem  AncestorBlock=NG_Genset_lib/Generator
  Modbus device : rtio_generic_modbus/Modbus device  conf_name=CHP_slave_cfg.opal  conf_name_mask=CHP_slave_cfg.xls  sample_time=Ts
  Mux1 : Mux  Inputs=5
  A : PMIOPort  Tag=A  Port=1  Side=Right
      settings: AttributesFormatString=A
  B : PMIOPort  Port=2  Side=Right
  C : PMIOPort  Port=3  Side=Right
  Out1 : Outport
  Out2 : Outport  Port=2
  Generator Data : Outport  Port=3
  GCB Control : Outport  Port=4
  wires:
  In2/1 -> CHPThermalModel/5  "CHP_SIM_Cmds"
  Generator/1(Digital Inputs) -> Out2/1
  Bus Creator2/1 -> Out1/1, Bus Selector7/1  "CHPData"
  Bus Selector6/1 -> CHPThermalModel/1  "<Heat Recovered; MBtu/hr>"
  Generator/4(1 LCB Control (opt)) -> [Load1_opt]
  Generator/3(Gen1 GCB Control) -> GCB Control/1
  MCB/1 -> Generator/6(MCB1 V and I)
  Generator/5(2 LCB Control (opt)) -> [Load2_opt]
  Manual Control (opt)/1 -> Generator/4(Manual Control Gen1 (opt))
  GCB/1 -> Generator/5(GCB1 V and I)
  Generator/2(Gen1 Monitor) -> Generator Data/1
  Woodward Enable/1 -> Generator/3(Woodward Enable)
  Modbus device/2 -> Demux/1
  Generator/8(Out2) -> Bus Selector6/1, Bus Creator2/2  "Thermal data"
  CHPThermalModel/3 -> Bus Creator2/4
  Demux/1 -> CHPThermalModel/3
  Mux1/1 -> Modbus device/4
  In1/1 -> CHPThermalModel/2
  Bus Selector7/1 -> Mux1/1  "<TempActual>"
  Bus Selector7/4 -> Mux1/4  "<Heat Recovered; MBtu/hr>"
  Bus Selector7/5 -> Mux1/5  "<CO2 lbm/hr>"
  Bus Selector7/2 -> Mux1/2  "<HeatFromBoiler MBtu/hr>"
  Digital Outputs/1 -> Generator/1(Digital Outputs)
  Generator/7(Grid Control (opt)) -> [Grid_opt]
  Console Breakers/1 -> Generator/2(Console Breakers)
  Generator/6(Gen 1 MCB Control (opt)) -> [Mains1_opt]
  CHPThermalModel/2 -> Bus Creator2/3
  Demux/2 -> CHPThermalModel/4
  CHPThermalModel/1 -> Bus Creator2/1  "TempActual"
  Bus Selector7/3 -> Mux1/3  "<CHPHeatContribution MBtu/hr>"
  connections:
  Generator/RConn1 -- A/RConn1
  Generator/RConn2 -- B/RConn1
  Generator/RConn3 -- C/RConn1

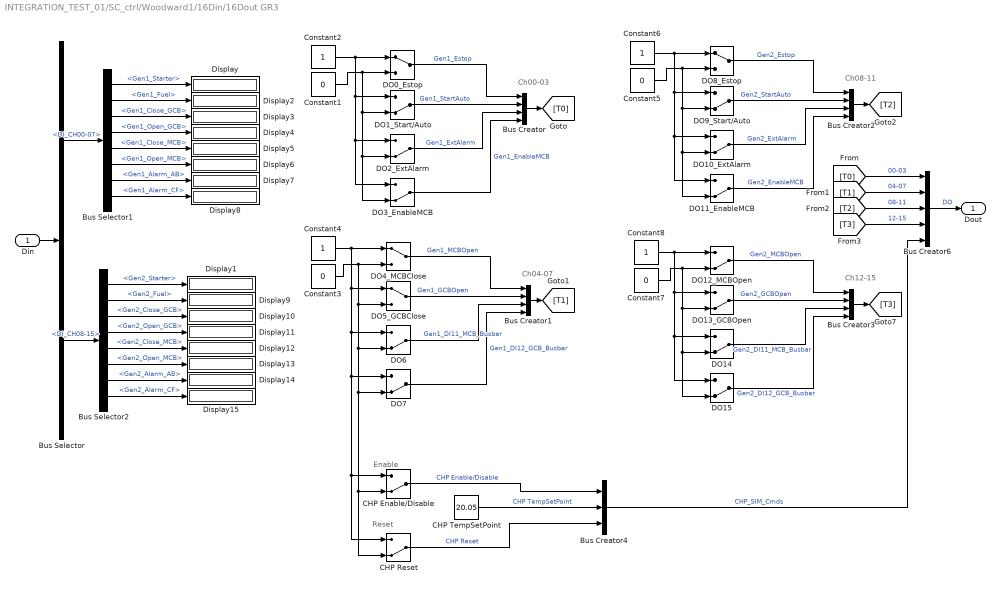
== system INTEGRATION_TEST_01/SC_ctrl/Woodward1/16Din/16Dout GR3 ==
  note: Reset
  note: Enable
  note: Ch12-15
  note: Ch08-11
  note: Ch04-07
  note: Ch00-03
  Din : Inport
  Bus Creator{,1..3} (4 alike) : BusCreator
  Bus Creator4 : BusCreator  Inputs=3
  Bus Creator6 : BusCreator  Inputs=5
  Bus Selector : BusSelector  OutputSignals=DIN.DI_CH00-07,DIN.DI_CH08-15
  Bus Selector1 : BusSelector  OutputSignals=Gen1_Starter,Gen1_Fuel,Gen1_Close_GCB,Gen1_Open_GCB,Gen1_Close_MCB,Gen1_Open_MCB,Gen1_Alarm_AB,Gen1_Alarm_CF
  Bus Selector2 : BusSelector  OutputSignals=Gen2_Starter,Gen2_Fuel,Gen2_Close_GCB,Gen2_Open_GCB,Gen2_Close_MCB,Gen2_Open_MCB,Gen2_Alarm_AB,Gen2_Alarm_CF
  CHP Enable/Disable : ManualSwitch  CurrentSetting=0
  CHP Reset : ManualSwitch  CurrentSetting=0
  CHP TempSetPoint : Constant  Value=20.05
  Constant{1,3,5,7} (4 alike) : Constant  Value=0
  Constant{2,4,6,8} (4 alike) : Constant
  DO0_Estop : ManualSwitch
  DO10_ExtAlarm : ManualSwitch  CurrentSetting=0
  DO11_EnableMCB : ManualSwitch  CurrentSetting=0
  DO12_MCBOpen : ManualSwitch  CurrentSetting=0
  DO13_GCBOpen : ManualSwitch  CurrentSetting=0
  DO{6..7,14..15} (4 alike) : ManualSwitch  CurrentSetting=0
  DO1_Start/Auto : ManualSwitch  CurrentSetting=0
  DO2_ExtAlarm : ManualSwitch  CurrentSetting=0
  DO3_EnableMCB : ManualSwitch  CurrentSetting=0
  DO4_MCBClose : ManualSwitch
  DO5_GCBClose : ManualSwitch
  DO8_Estop : ManualSwitch
  DO9_Start/Auto : ManualSwitch  CurrentSetting=0
  Display{,1..15} (16 alike) : Display
  Dout : Outport
  wires:
  Bus Selector1/7 -> Display7/1  "<Gen1_Alarm_AB>"
  Bus Selector1/4 -> Display4/1  "<Gen1_Open_GCB>"
  Bus Selector2/8 -> Display15/1  "<Gen2_Alarm_CF>"
  Bus Selector2/7 -> Display14/1  "<Gen2_Alarm_AB>"
  Bus Selector2/6 -> Display13/1  "<Gen2_Open_MCB>"
  Bus Selector2/5 -> Display12/1  "<Gen2_Close_MCB>"
  Bus Selector2/4 -> Display11/1  "<Gen2_Open_GCB>"
  Bus Selector2/3 -> Display10/1  "<Gen2_Close_GCB>"
  Bus Selector2/2 -> Display9/1  "<Gen2_Fuel>"
  Bus Selector2/1 -> Display1/1  "<Gen2_Starter>"
  Bus Selector/2 -> Bus Selector2/1  "<DI_CH08-15>"
  Bus Selector1/8 -> Display8/1  "<Gen1_Alarm_CF>"
  Bus Selector1/6 -> Display6/1  "<Gen1_Open_MCB>"
  Bus Selector1/5 -> Display5/1  "<Gen1_Close_MCB>"
  Bus Selector1/3 -> Display3/1  "<Gen1_Close_GCB>"
  Bus Selector1/2 -> Display2/1  "<Gen1_Fuel>"
  Bus Selector1/1 -> Display/1  "<Gen1_Starter>"
  Bus Selector/1 -> Bus Selector1/1  "<DI_CH00-07>"
  Din/1 -> Bus Selector/1
  [T3] -> Bus Creator6/4  "12-15"
  [T2] -> Bus Creator6/3  "08-11"
  [T1] -> Bus Creator6/2  "04-07"
  [T0] -> Bus Creator6/1  "00-03"
  Bus Creator2/1 -> [T2]
  Bus Creator3/1 -> [T3]
  Bus Creator1/1 -> [T1]
  Bus Creator/1 -> [T0]
  DO15/1 -> Bus Creator3/4  "Gen2_DI12_GCB_Busbar"
  DO14/1 -> Bus Creator3/3  "Gen2_DI11_MCB_Busbar"
  DO13_GCBOpen/1 -> Bus Creator3/2  "Gen2_GCBOpen"
  DO12_MCBOpen/1 -> Bus Creator3/1  "Gen2_MCBOpen"
  Constant7/1 -> DO12_MCBOpen/2, DO13_GCBOpen/2, DO15/2, DO14/2
  Constant8/1 -> DO12_MCBOpen/1, DO13_GCBOpen/1, DO15/1, DO14/1
  DO11_EnableMCB/1 -> Bus Creator2/4  "Gen2_EnableMCB"
  DO10_ExtAlarm/1 -> Bus Creator2/3  "Gen2_ExtAlarm"
  DO9_Start/Auto/1 -> Bus Creator2/2  "Gen2_StartAuto"
  DO8_Estop/1 -> Bus Creator2/1  "Gen2_Estop"
  Constant5/1 -> DO10_ExtAlarm/2, DO11_EnableMCB/2, DO9_Start/Auto/2, DO8_Estop/2
  Constant6/1 -> DO10_ExtAlarm/1, DO11_EnableMCB/1, DO9_Start/Auto/1, DO8_Estop/1
  DO7/1 -> Bus Creator1/4  "Gen1_DI12_GCB_Busbar"
  DO6/1 -> Bus Creator1/3  "Gen1_DI11_MCB_Busbar"
  DO5_GCBClose/1 -> Bus Creator1/2  "Gen1_GCBOpen"
  DO4_MCBClose/1 -> Bus Creator1/1  "Gen1_MCBOpen"
  Constant3/1 -> DO4_MCBClose/2, DO5_GCBClose/2, DO7/2, CHP Reset/2, CHP Enable/Disable/2, DO6/2
  Constant4/1 -> DO4_MCBClose/1, DO5_GCBClose/1, CHP Reset/1, CHP Enable/Disable/1, DO7/1, DO6/1
  DO3_EnableMCB/1 -> Bus Creator/4  "Gen1_EnableMCB"
  DO2_ExtAlarm/1 -> Bus Creator/3  "Gen1_ExtAlarm"
  DO1_Start/Auto/1 -> Bus Creator/2  "Gen1_StartAuto"
  DO0_Estop/1 -> Bus Creator/1  "Gen1_Estop"
  Constant1/1 -> DO2_ExtAlarm/2, DO3_EnableMCB/2, DO1_Start/Auto/2, DO0_Estop/2
  Constant2/1 -> DO2_ExtAlarm/1, DO3_EnableMCB/1, DO1_Start/Auto/1, DO0_Estop/1
  Bus Creator6/1 -> Dout/1  "DO"
  CHP Enable/Disable/1 -> Bus Creator4/1  "CHP Enable/Disable"
  CHP TempSetPoint/1 -> Bus Creator4/2  "CHP TempSetPoint"
  CHP Reset/1 -> Bus Creator4/3  "CHP Reset"
  Bus Creator4/1 -> Bus Creator6/5  "CHP_SIM_Cmds"

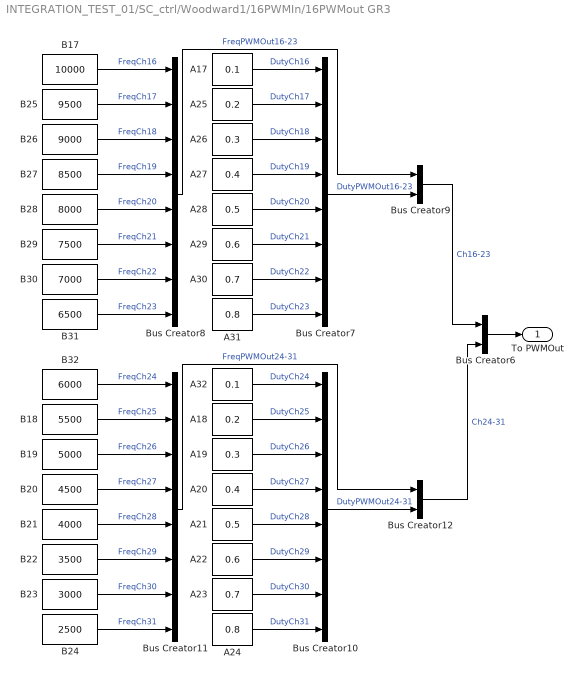
== system INTEGRATION_TEST_01/SC_ctrl/Woodward1/16PWMIn/16PWMout GR3 ==
  A17 : Constant  Value=0.1
  A18 : Constant  Value=0.2
  A19 : Constant  Value=0.3
  A20 : Constant  Value=0.4
  A21 : Constant  Value=0.5
  A22 : Constant  Value=0.6
  A23 : Constant  Value=0.7
  A24 : Constant  Value=0.8
  A25 : Constant  Value=0.2
  A26 : Constant  Value=0.3
  A27 : Constant  Value=0.4
  A28 : Constant  Value=0.5
  A29 : Constant  Value=0.6
  A30 : Constant  Value=0.7
  A31 : Constant  Value=0.8
  A32 : Constant  Value=0.1
  B17 : Constant  Value=10000
  B18 : Constant  Value=5500
  B19 : Constant  Value=5000
  B20 : Constant  Value=4500
  B21 : Constant  Value=4000
  B22 : Constant  Value=3500
  B23 : Constant  Value=3000
  B24 : Constant  Value=2500
  B25 : Constant  Value=9500
  B26 : Constant  Value=9000
  B27 : Constant  Value=8500
  B28 : Constant  Value=8000
  B29 : Constant  Value=7500
  B30 : Constant  Value=7000
  B31 : Constant  Value=6500
  B32 : Constant  Value=6000
  Bus Creator{7..8,10..11} (4 alike) : BusCreator  Inputs=8
  Bus Creator12 : BusCreator  Inputs=2
  Bus Creator6 : BusCreator  Inputs=2
  Bus Creator9 : BusCreator  Inputs=2
  To PWMOut : Outport
  wires:
  Bus Creator9/1 -> Bus Creator6/1  "Ch16-23"
  Bus Creator12/1 -> Bus Creator6/2  "Ch24-31"
  Bus Creator11/1 -> Bus Creator12/1  "FreqPWMOut24-31"
  Bus Creator10/1 -> Bus Creator12/2  "DutyPWMOut24-31"
  B24/1 -> Bus Creator11/8  "FreqCh31"
  B23/1 -> Bus Creator11/7  "FreqCh30"
  B22/1 -> Bus Creator11/6  "FreqCh29"
  B21/1 -> Bus Creator11/5  "FreqCh28"
  B20/1 -> Bus Creator11/4  "FreqCh27"
  B19/1 -> Bus Creator11/3  "FreqCh26"
  B18/1 -> Bus Creator11/2  "FreqCh25"
  B32/1 -> Bus Creator11/1  "FreqCh24"
  A24/1 -> Bus Creator10/8  "DutyCh31"
  A23/1 -> Bus Creator10/7  "DutyCh30"
  A22/1 -> Bus Creator10/6  "DutyCh29"
  A21/1 -> Bus Creator10/5  "DutyCh28"
  A20/1 -> Bus Creator10/4  "DutyCh27"
  A19/1 -> Bus Creator10/3  "DutyCh26"
  A18/1 -> Bus Creator10/2  "DutyCh25"
  A32/1 -> Bus Creator10/1  "DutyCh24"
  Bus Creator8/1 -> Bus Creator9/1  "FreqPWMOut16-23"
  Bus Creator7/1 -> Bus Creator9/2  "DutyPWMOut16-23"
  B31/1 -> Bus Creator8/8  "FreqCh23"
  B30/1 -> Bus Creator8/7  "FreqCh22"
  B29/1 -> Bus Creator8/6  "FreqCh21"
  B28/1 -> Bus Creator8/5  "FreqCh20"
  B27/1 -> Bus Creator8/4  "FreqCh19"
  B26/1 -> Bus Creator8/3  "FreqCh18"
  B25/1 -> Bus Creator8/2  "FreqCh17"
  B17/1 -> Bus Creator8/1  "FreqCh16"
  A31/1 -> Bus Creator7/8  "DutyCh23"
  A30/1 -> Bus Creator7/7  "DutyCh22"
  A29/1 -> Bus Creator7/6  "DutyCh21"
  A28/1 -> Bus Creator7/5  "DutyCh20"
  A27/1 -> Bus Creator7/4  "DutyCh19"
  A26/1 -> Bus Creator7/3  "DutyCh18"
  A25/1 -> Bus Creator7/2  "DutyCh17"
  A17/1 -> Bus Creator7/1  "DutyCh16"
  Bus Creator6/1 -> To PWMOut/1

== system INTEGRATION_TEST_01/SC_ctrl/Woodward1/16TSDIn/16 TSDOut GR3 ==
  Bus Creator1 : BusCreator  Inputs=3
  Din/Dout ch16-23 : Subsystem
  Din/Dout ch24-31 : Subsystem
  Dout state ctrl : Subsystem
  TSDout : Outport
  wires:
  Bus Creator1/1 -> TSDout/1
  Dout state ctrl/1(Event State OUT) -> Bus Creator1/3  "states"
  Din/Dout ch16-23/1(Out1) -> Bus Creator1/1  "times CH16-23"
  Din/Dout ch24-31/1(Out1) -> Bus Creator1/2  "times CH24-31"

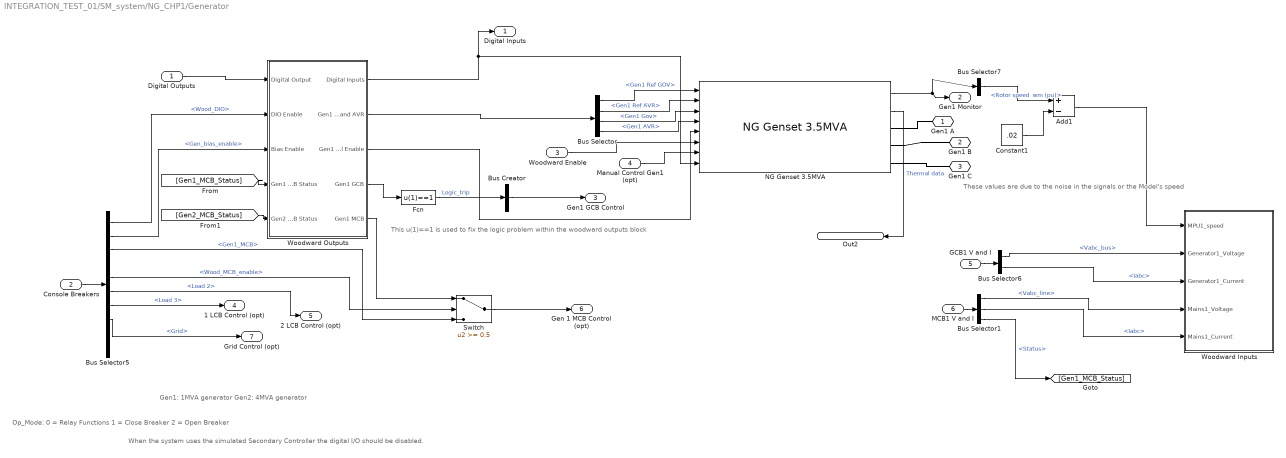
== system INTEGRATION_TEST_01/SM_system/NG_CHP1/Generator ==
  note: Op_Mode:
      | 0 = Relay Functions
      | 1 = Close Breaker
      | 2 = Open Breaker
  note: These values are due to
      | the noise in the signals
      | or the Model's speed
  note: Gen1: 1MVA generator
      | Gen2: 4MVA generator
  note: When the system uses the simulated
      | Secondary Controller the digital I/O
      | should be disabled.
  note: This u(1)==1 is used to fix the logic problem within the woodward outputs block
  Digital Outputs : Inport
  Console Breakers : Inport  Port=2
  Woodward Enable : Inport  Port=3
  Manual Control Gen1 (opt) : Inport  Port=4
  GCB1 V and I : Inport  Port=5
  MCB1 V and I : Inport  Port=6
  Add1 : Sum  Inputs=+-
  Bus Creator : BusCreator  Inputs=1
  Bus Selector : BusSelector  OutputSignals=Gen1 Ref GOV,Gen1 Ref AVR,Gen1 Gov,Gen1 AVR
  Bus Selector1 : BusSelector  OutputSignals=Vabc_line,Iabc,Status
  Bus Selector5 : BusSelector  OutputSignals=Wood_DIO,Gen_bias_enable,Gen1_MCB,Gen2_MCB,Wood_MCB_enable,Load 2,Load 3,Grid,Gen2_enable,Load 1
  Bus Selector6 : BusSelector  OutputSignals=Vabc_bus,Iabc
  Bus Selector7 : BusSelector  OutputSignals="w.w.Rotor speed  wm (pu)"
  Constant1 : Constant  Value=.02
  Fcn : Fcn  Expr=u(1)==1
  NG Genset 3.5MVA : NG_Genset_lib/NG Genset 3.5MVA  control_mode=1
  Switch : Switch  Threshold=0.5
  Woodward Inputs : Subsystem
  Woodward Outputs : Subsystem
  Gen1 A : PMIOPort  Port=1  Side=Right
  Gen1 B : PMIOPort  Port=2  Side=Right
  Gen1 C : PMIOPort  Port=3  Side=Right
  Digital Inputs : Outport
  Gen1 Monitor : Outport  Port=2
  Gen1 GCB Control : Outport  Port=3
  1 LCB Control (opt) : Outport  Port=4
  2 LCB Control (opt) : Outport  Port=5
  Gen 1 MCB Control (opt) : Outport  Port=6
  Grid Control (opt) : Outport  Port=7
  Out2 : Outport  Port=8
  wires:
  Fcn/1 -> Bus Creator/1  "Logic_trip"
  Bus Creator/1 -> Gen1 GCB Control/1
  NG Genset 3.5MVA/1 -> Bus Selector7/1, Gen1 Monitor/1
  Bus Selector6/1 -> Woodward Inputs/2(Generator1_Voltage)  "<Vabc_bus>"
  Bus Selector6/2 -> Woodward Inputs/3(Generator1_Current)  "<Iabc>"
  Bus Selector5/1 -> Woodward Outputs/2(DIO Enable)  "<Wood_DIO>"
  Manual Control Gen1 (opt)/1 -> NG Genset 3.5MVA/7
  Bus Selector5/2 -> Woodward Outputs/3(Bias Enable)  "<Gen_bias_enable>"
  Bus Selector7/1 -> Add1/1  "<Rotor speed  wm (pu)>"
  Woodward Enable/1 -> NG Genset 3.5MVA/6
  Woodward Outputs/3(Gen1 Fuel Enable) -> NG Genset 3.5MVA/5
  Bus Selector5/5 -> Switch/2  "<Wood_MCB_enable>"
  Woodward Outputs/5(Gen1 MCB) -> Switch/1
  Digital Outputs/1 -> Woodward Outputs/1(Digital Output)
  GCB1 V and I/1 -> Bus Selector6/1
  Woodward Outputs/4(Gen1 GCB) -> Fcn/1
  Console Breakers/1 -> Bus Selector5/1
  Bus Selector5/7 -> 1 LCB Control (opt)/1  "<Load 3>"
  Switch/1 -> Gen 1 MCB Control (opt)/1
  MCB1 V and I/1 -> Bus Selector1/1
  Bus Selector1/1 -> Woodward Inputs/4(Mains1_Voltage)  "<Vabc_line>"
  Bus Selector1/2 -> Woodward Inputs/5(Mains1_Current)  "<Iabc>"
  Woodward Outputs/2(Gen1 Gov and AVR) -> Bus Selector/1
  Bus Selector/1 -> NG Genset 3.5MVA/1  "<Gen1 Ref GOV>"
  Bus Selector/2 -> NG Genset 3.5MVA/2  "<Gen1 Ref AVR>"
  Bus Selector/3 -> NG Genset 3.5MVA/3  "<Gen1 Gov>"
  Bus Selector/4 -> NG Genset 3.5MVA/4  "<Gen1 AVR>"
  Bus Selector1/3 -> [Gen1_MCB_Status]  "<Status>"
  [Gen1_MCB_Status] -> Woodward Outputs/4(Gen1 MCB Status)
  [Gen2_MCB_Status] -> Woodward Outputs/5(Gen2 MCB Status)
  Bus Selector5/6 -> 2 LCB Control (opt)/1  "<Load 2>"
  Bus Selector5/3 -> Switch/3  "<Gen1_MCB>"
  Bus Selector5/8 -> Grid Control (opt)/1  "<Grid>"
  Constant1/1 -> Add1/2
  NG Genset 3.5MVA/2 -> Out2/1  "Thermal data"
  Add1/1 -> Woodward Inputs/1(MPU1_speed)
  Woodward Outputs/1(Digital Inputs) -> Digital Inputs/1, NG Genset 3.5MVA/8
  connections:
  NG Genset 3.5MVA/RConn1 -- Gen1 A/RConn1
  NG Genset 3.5MVA/RConn2 -- Gen1 B/RConn1
  NG Genset 3.5MVA/RConn3 -- Gen1 C/RConn1

== system INTEGRATION_TEST_01/SC_ctrl/Woodward1/16TSDIn/16 TSDOut GR3/Din/Dout ch16-23 ==
  Bus Creator3 : BusCreator  Inputs=8
  times17 : Constant  Value=[0.05 0.15 0.25 0.35]
  times18 : Constant  Value=[0.1 0.2 0.3 0.4]
  times19 : Constant  Value=[0.15 0.25 0.35 0.45]
  times20 : Constant  Value=[0.2 0.3 0.4 0.5]
  times21 : Constant  Value=[0.25 0.35 0.45 0.55]
  times22 : Constant  Value=[0.3 0.4 0.5 0.6]
  times23 : Constant  Value=[0.3 0.4 0.5 0.6]
  times24 : Constant  Value=[0 0.1 0.2 0.3]
  Out1 : Outport
  wires:
  times24/1 -> Bus Creator3/1  "times17"
  times17/1 -> Bus Creator3/2  "times18"
  times18/1 -> Bus Creator3/3  "times19"
  times19/1 -> Bus Creator3/4  "times20"
  times20/1 -> Bus Creator3/5  "times21"
  times21/1 -> Bus Creator3/6  "times22"
  times22/1 -> Bus Creator3/7  "times23"
  times23/1 -> Bus Creator3/8  "times24"
  Bus Creator3/1 -> Out1/1

== system INTEGRATION_TEST_01/SC_ctrl/Woodward1/16TSDIn/16 TSDOut GR3/Din/Dout ch24-31 ==
  Bus Creator4 : BusCreator  Inputs=8
  times25 : Constant  Value=[0.05 0.15 0.25 0.35]
  times26 : Constant  Value=[0.1 0.2 0.3 0.4]
  times27 : Constant  Value=[0.15 0.25 0.35 0.45]
  times28 : Constant  Value=[0.2 0.3 0.4 0.5]
  times29 : Constant  Value=[0.25 0.35 0.45 0.55]
  times30 : Constant  Value=[0.3 0.4 0.5 0.6]
  times31 : Constant  Value=[0.3 0.4 0.5 0.6]
  times32 : Constant  Value=[0 0.1 0.2 0.3]
  Out1 : Outport
  wires:
  times32/1 -> Bus Creator4/1  "times25"
  times25/1 -> Bus Creator4/2  "times26"
  times26/1 -> Bus Creator4/3  "times27"
  times27/1 -> Bus Creator4/4  "times28"
  times28/1 -> Bus Creator4/5  "times29"
  times29/1 -> Bus Creator4/6  "times30"
  times30/1 -> Bus Creator4/7  "times31"
  times31/1 -> Bus Creator4/8  "times32"
  Bus Creator4/1 -> Out1/1

== system INTEGRATION_TEST_01/SC_ctrl/Woodward1/16TSDIn/16 TSDOut GR3/Dout state ctrl ==
  Bus Creator : BusCreator  Inputs=2
  Dout_CH16_CH23 : Subsystem
  Dout_CH24_CH31 : Subsystem
  Event State OUT : Outport
  wires:
  Bus Creator/1 -> Event State OUT/1
  Dout_CH16_CH23/1(Dout_CH8_CH15) -> Bus Creator/1  "CH16-23"
  Dout_CH24_CH31/1(Dout_CH8_CH15) -> Bus Creator/2  "CH24-31"
